simulink model "biomasa"  (R2016b)
settings: Solver=VariableStepAuto  StartTime=0.0  StopTime=10.0  RelTol=1e-3
values from neighbouring files (symbols this model uses):
  a = 0.01    [eu.m]    (also in matlab.mat)
  b = 0.2    [eu.m]    (also in matlab.mat)
  h = 0.2    [eu.m]    (also in matlab.mat)
  mu = 0.1    [eu.m]    (also in matlab.mat)
undefined symbols (not defined in the file or in its folder): K, r
libraries: simulink x1
settings Model: Creator=Asus  LastModifiedBy=Asus

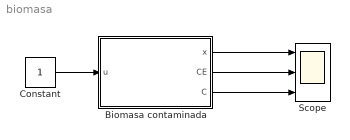
== system biomasa ==
  Biomasa contaminada : Subsystem  mask{par=0, x0=0}
      mask prompts: par "[r, K, a, b, h, mu]"; x0 "Condiciones iniciales"
      mask Display: image('D:\Dropbox\Ingeniería Matemática\Cuarto semestre\Monitoría lógica\imagen.jpg');
  Constant : Constant
  Scope : Scope  NumInputPorts=3
  wires:
  Constant/1 -> Biomasa contaminada/1(u)
  Biomasa contaminada/1(x) -> Scope/1
  Biomasa contaminada/2(CE) -> Scope/2
  Biomasa contaminada/3(C) -> Scope/3

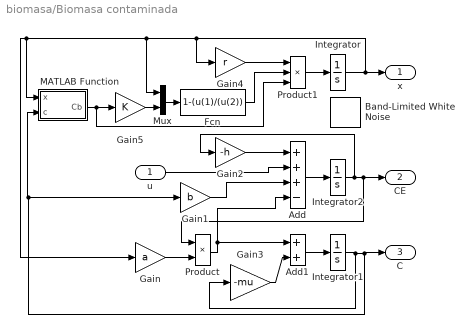
== system biomasa/Biomasa contaminada ==
  u : Inport
  Add : Sum  Inputs=+++-
  Add1 : Sum
  Band-Limited White Noise : simulink/Sources/Band-Limited White Noise  Cov=0.02  Ts=0  seed=[4000]
  Fcn : Fcn  Expr=1-(u(1)/(u(2))
  Gain : Gain  Gain=a
  Gain1 : Gain  Gain=b
  Gain2 : Gain  Gain=-h
  Gain3 : Gain  Gain=-mu
  Gain4 : Gain  Gain=r
  Gain5 : Gain  Gain=K
  Integrator : Integrator  InitialCondition=x0
  Integrator1 : Integrator  InitialCondition=x0
  Integrator2 : Integrator  InitialCondition=x0
  MATLAB Function : MATLAB Function  TreatAsAtomicUnit=on
  Mux : Mux  Inputs=2
  Product : Product
  Product1 : Product  Inputs=3
  x : Outport
  CE : Outport  Port=2
  C : Outport  Port=3
  wires:
  Product/1 -> Add/4, Add1/1
  Gain3/1 -> Add1/2
  Gain1/1 -> Add/3
  Gain4/1 -> Product1/1
  MATLAB Function/1(Cb) -> Gain5/1, Product1/3
  Product1/1 -> Integrator/1
  Integrator/1 -> Gain4/1, Mux/1, MATLAB Function/1(x), Gain/1, x/1
  Add1/1 -> Integrator1/1
  Integrator1/1 -> Gain3/1, Gain1/1, MATLAB Function/2(c), C/1
  Gain5/1 -> Mux/2
  Mux/1 -> Fcn/1
  Fcn/1 -> Product1/2
  u/1 -> Add/2
  Gain2/1 -> Add/1
  Add/1 -> Integrator2/1
  Integrator2/1 -> Gain2/1, Product/1, CE/1
  Gain/1 -> Product/2

== matlab function biomasa/Biomasa contaminada/MATLAB Function ==
  data: x input; c input; Cb output
function Cb = fcn(x, c)
if x == 0
    Cb = 0;
else
    Cb = c/x;
end
end
